simulink library "Library_Betriebsstrategie"  (R2018b)
settings: Solver=VariableStepAuto  StartTime=0.0  StopTime=10.0  RelTol=1e-3  EnableMultiTasking=on
undefined symbols (not defined in the file): akt_eUELG_HA, akt_eUELG_VA, akt_keinMVS_HA, akt_keinMVS_VA, akt_LSD_HA, akt_LSD_VA, akt_mUELG_HA, akt_mUELG_VA, akt_OD_HA, akt_OD_VA, DiscIntNeverNeededParam, magnitude, mu_road, mu_road_LF, mu_road_LR, mu_road_RF, mu_road_RR, par_MDT, par_VEH, stepsize
libraries: simulink x13
(part 4 of 6)

== system Library_Betriebsstrategie/Momentverteilung_LR/Gierrate Referenz Berechnung ==
  note: Gewünschte Gierrate nach:
      | psip_desired = vx * delta / (l + vx^2 * K_us )
  note: Limit für die Gierrate
  input : Inport
  delta_wheel : Inport  Port=2
  FZG parameter : Inport  Port=3
  2 Räder : Constant  Value=0.5
  Abs : Abs
  Abs1 : Abs
  Add : Sum
  Add1 : Sum  Inputs=+--
  Add2 : Sum
  Bus Selector : BusSelector  OutputSignals=l,g
  Bus Selector1 : BusSelector  OutputSignals=delta_RF,delta_LF
  Bus Selector2 : BusSelector  OutputSignals=x.ax,beta.beta,beta.betap,x.vx
  Constant20 : Constant  Value=mu_road
  Divide : Product  Inputs=*/
  Divide1 : Product  Inputs=**/
  Divide2 : Product  Inputs=**/
  Divide3 : Product  Inputs=*/
  Kus : Constant  Value=0
  Product : Product
  Product1 : Product
  Product2 : Product
  Sicherheitsfaktor : Gain  Gain=0.90
  Sign : Signum
  Sqrt : Sqrt  SaturateOnIntegerOverflow=on
  Sum : Sum  Inputs=|++
  delta mittel : Product
  eins : Constant
  min : MinMax  Inputs=2
  tan (beta) : Trigonometry  Operator=tan
  tan^2 (beta) : Math  Operator=square  SaturateOnIntegerOverflow=on
  vx^2 : Math  Operator=square  SaturateOnIntegerOverflow=on
  Gierrate ref : Outport
  wires:
  FZG parameter/1 -> Bus Selector/1
  Product/1 -> Divide/1
  Bus Selector/1 -> Sum/2  "<l>"
  vx^2/1 -> Product1/1
  Sum/1 -> Divide/2
  Product1/1 -> Sum/1
  Kus/1 -> Product1/2
  Divide/1 -> Abs/1  "Gierrate gewuenscht"
  delta_wheel/1 -> Bus Selector1/1
  Bus Selector1/1 -> Add/1  "<delta_RF>"
  Bus Selector1/2 -> Add/2  "<delta_LF>"
  Add/1 -> delta mittel/1
  2 Räder/1 -> delta mittel/2
  delta mittel/1 -> Sign/1, Product/2
  input/1 -> Bus Selector2/1
  Bus Selector2/4 -> Divide2/3, Divide1/3, vx^2/1, Product/1  "<vx>"
  Sicherheitsfaktor/1 -> Abs1/1  "Gierrate Limit"
  Add1/1 -> Sicherheitsfaktor/1
  Sign/1 -> Product2/1  "Vorzeichen von delta"
  min/1 -> Product2/2
  Product2/1 -> Gierrate ref/1
  Abs/1 -> min/1
  Abs1/1 -> min/2
  Divide1/1 -> Add1/1
  Bus Selector/2 -> Divide1/2  "<g>"
  Constant20/1 -> Divide1/1
  Divide2/1 -> Add1/2
  Bus Selector2/1 -> Divide2/2  "<ax>"
  tan (beta)/1 -> tan^2 (beta)/1, Divide2/1
  Bus Selector2/2 -> tan (beta)/1  "<beta>"
  Divide3/1 -> Add1/3
  Bus Selector2/3 -> Divide3/1  "<betap>"
  tan^2 (beta)/1 -> Add2/1
  eins/1 -> Add2/2
  Add2/1 -> Sqrt/1
  Sqrt/1 -> Divide3/2

== system Library_Betriebsstrategie/Momentverteilung_LR/Momente für die Reibbremse ==
  M_antr : Inport
  M_wheel : Inport  Port=2
  v_x : Inport  Port=3
  bkv : Inport  Port=4
  Add : Sum  Inputs=-+
  Add1 : Sum  Inputs=++++
  Bias : Bias  Bias=-1
  Bus Selector : BusSelector  OutputSignals=M_antr_LF,M_antr_LR,M_antr_RF,M_antr_RR
  Product4 : Product  Inputs=3
  Product5 : Product  Inputs=3
  Saturation2 : Saturate  UpperLimit=0  LowerLimit=-5000
  Sign : Signum
  Signal Conversion : SignalConversion  OverrideOpt=off
  Signal Conversion1 : SignalConversion  OverrideOpt=off
  Unary Minus : UnaryMinus
  Unit Delay2 : UnitDelay  InitialCondition=2  SampleTime=-1
  LF : Outport
  LR : Outport  Port=2
  RF : Outport  Port=3
  RR : Outport  Port=4
  wires:
  Add/1 -> Saturation2/1
  Saturation2/1 -> Product5/1, Product4/2
  Bias/1 -> Unary Minus/1
  Unary Minus/1 -> Product5/2
  Signal Conversion/1 -> LF/1  "M_brems_LF"
  Signal Conversion1/1 -> LR/1  "M_brems_LR"
  Product4/1 -> RF/1, Signal Conversion/1  "M_brems_RF"
  Product5/1 -> RR/1, Signal Conversion1/1  "M_brems_RR"
  Sign/1 -> Product4/3, Product5/3
  Unit Delay2/1 -> Sign/1
  bkv/1 -> Product4/1, Bias/1
  v_x/1 -> Unit Delay2/1
  M_wheel/1 -> Add/2
  M_antr/1 -> Bus Selector/1
  Bus Selector/4 -> Add1/4  "<M_antr_RR>"
  Bus Selector/3 -> Add1/3  "<M_antr_RF>"
  Bus Selector/2 -> Add1/2  "<M_antr_LR>"
  Bus Selector/1 -> Add1/1  "<M_antr_LF>"
  Add1/1 -> Add/1

== system Library_Betriebsstrategie/Momentverteilung_LR/Motor Limits ==
  Input : Inport
  Add{1..4} (4 alike) : Sum
  Bus Creator : BusCreator  Inputs=8
  Bus Selector : BusSelector  OutputSignals=omega
  Demux : Demux
  Demux1 : Demux
  Gain{,1..7} (8 alike) : Gain  Gain=0.5
  M_Antr : Lookup_n-D  NumberOfTableDimensions=1  BreakpointsForDimension1=par_VEH.dt_nmax/par_VEH.dt_i/60*2*pi  Table=par_VEH.dt_Mmax*par_VEH.dt_i/2  InternalRulePriority=Speed  RndMeth=Simplest  InputSameDT=on
  M_Reku : Lookup_n-D  NumberOfTableDimensions=1  BreakpointsForDimension1=par_VEH.dt_nmin/par_VEH.dt_i/60*2*pi  Table=par_VEH.dt_Mmin*par_VEH.dt_i/2  InternalRulePriority=Speed  RndMeth=Simplest  InputSameDT=on
  Rate Transition : RateTransition  OutPortSampleTime=stepsize*10
  Rate Transition1 : RateTransition  OutPortSampleTimeOpt=Inherit  OutPortSampleTime=0.001
  Rate Transition2 : RateTransition  OutPortSampleTime=stepsize*10
  Rate Transition3 : RateTransition  OutPortSampleTimeOpt=Inherit  OutPortSampleTime=0.001
  M_limit : Outport
  wires:
  Bus Creator/1 -> M_limit/1
  M_Reku/1 -> Rate Transition1/1
  Rate Transition/1 -> M_Reku/1
  M_Antr/1 -> Rate Transition3/1
  Rate Transition2/1 -> M_Antr/1
  Rate Transition1/1 -> Demux/1
  Demux/1 -> Add1/1
  Demux/2 -> Add1/2
  Add1/1 -> Gain4/1, Gain/1
  Demux/3 -> Add2/1
  Demux/4 -> Add2/2
  Add2/1 -> Gain5/1, Gain1/1
  Demux1/1 -> Add3/1
  Demux1/2 -> Add3/2
  Add3/1 -> Gain6/1, Gain2/1
  Demux1/3 -> Add4/1
  Demux1/4 -> Add4/2
  Add4/1 -> Gain7/1, Gain3/1
  Rate Transition3/1 -> Demux1/1
  Bus Selector/1 -> Rate Transition2/1, Rate Transition/1  "<omega>"
  Input/1 -> Bus Selector/1
  Gain1/1 -> Bus Creator/3  "M_RF_lb"
  Gain2/1 -> Bus Creator/5  "M_LF_ub"
  Gain3/1 -> Bus Creator/7  "M_RF_ub"
  Gain4/1 -> Bus Creator/1  "M_LF_lb"
  Gain/1 -> Bus Creator/2  "M_LR_lb"
  Gain5/1 -> Bus Creator/4  "M_RR_lb"
  Gain6/1 -> Bus Creator/6  "M_LR_ub"
  Gain7/1 -> Bus Creator/8  "M_RR_ub"

== system Library_Betriebsstrategie/Momentverteilung_LR/Radmomentenaufteilung ==
  note: Optimale Distribution Factors
  note: Momentenverteilung
  note: Aufbringen des TV-Moments
  Input : Inport
  M_wheel : Inport  Port=2
  M_z_desired : Inport  Port=3
  FZG parameter : Inport  Port=4
  Bias : Bias  Bias=-1
  Bias1 : Bias  Bias=-1
  Bus Selector : BusSelector  OutputSignals=sF05,r_eff_F
  Divide : Product  Inputs=*/
  Divide1 : Product  Inputs=*/
  Gain : Gain  Gain=0.5
  Optimierung links : Subsystem
  Optimierung rechts : Subsystem
  Product{,1..5} (6 alike) : Product
  Scope2 : Scope  NumInputPorts=4
  Sum : Sum  Inputs=|++
  Sum1 : Sum  Inputs=|+-
  Unary Minus : UnaryMinus
  Unary Minus1 : UnaryMinus
  r_stat0 : Constant  Value=par_VEH.r_stat0
  sF05 : Constant  Value=par_VEH.sF05
  M_antr_LF : Outport
  M_antr_LR : Outport  Port=2
  M_antr_RF : Outport  Port=3
  M_antr_RR : Outport  Port=4
  wires:
  M_wheel/1 -> Divide/1
  M_z_desired/1 -> Divide1/1
  Divide/1 -> Sum1/1, Sum/1  "F_x"
  Divide1/1 -> Sum1/2, Sum/2
  Sum1/1 -> Product/1
  Gain/1 -> Product1/2, Product/2
  Sum/1 -> Product1/1
  Product/1 -> Optimierung links/1(M_wheel_left), Product5/2, Product3/1  "M_wheel_left"
  Product1/1 -> Optimierung rechts/2(M_wheel_right), Product2/1, Product4/2  "M_wheel_right"
  Product3/1 -> Scope2/1, M_antr_LF/1  "M_LF"
  Product4/1 -> M_antr_RR/1, Scope2/4  "M_RR"
  Product5/1 -> Scope2/2, M_antr_LR/1  "M_LR"
  Optimierung rechts/1(gamma_right) -> Bias1/1, Product2/2
  r_stat0/1 -> Divide/2, Gain/1
  sF05/1 -> Divide1/2
  Product2/1 -> Scope2/3, M_antr_RF/1  "M_RF"
  Input/1 -> Optimierung links/2(Input), Optimierung rechts/1(Input)
  FZG parameter/1 -> Bus Selector/1
  Bias/1 -> Unary Minus/1
  Optimierung links/1(gamma_left) -> Bias/1, Product3/2
  Unary Minus/1 -> Product5/1
  Bias1/1 -> Unary Minus1/1
  Unary Minus1/1 -> Product4/1

== system Library_Betriebsstrategie/Momentverteilung_LR/Reifen Limits ==
  note: Kammscher Kreis liefert mit aktuellen mue und F_z_i die limits für Fx
  ParVehicle : Inport
  Fx_limits : Outport

== system Library_Betriebsstrategie/Momentverteilung_LR1/Feedback Controller ==
  note: Sigmoid Funktion
  note: M_z punkt = - Iz * K * sign(sigma - 1/2sigma(Tc))
  note: 1/2 sigma(Tc)
  Gierrate : Inport
  Gierrate ref : Inport  Port=2
  Iz : Inport  Port=3
  -1 : Gain  Gain=-1
  Abs : Abs
  Add : Sum
  Discrete D : simulink/Discrete/Discrete Derivative  gainval=1.0  ICPrevScaledInput=0.0  OutMin=[]  OutMax=[]  OutDataType=fixdt(1, 16)  OutScaling=2^-10  DoSatur=off
  Discrete-Time Integrator : DiscreteIntegrator  SampleTime=0.1  ICPrevOutput=DiscIntNeverNeededParam  ICPrevScaledInput=DiscIntNeverNeededParam
  Divide : Product  Inputs=*/
  Divide1 : Product  Inputs=*/
  Einheitenkorrektur : Constant  Value=1000
  Gain : Gain  Gain=0.5
  K : Gain  Gain=8
  Memory : Memory  LinearizeAsDelay=on
  Product : Product
  Sum : Sum  Inputs=|-+
  Sum1 : Sum  Inputs=|+-
  Unit Delay : UnitDelay  SampleTime=0.1
  Zero Crossing : Subsystem
  epsilon : Constant  Value=0.015
  M_z_desired : Outport
  wires:
  Divide1/1 -> Product/2
  Einheitenkorrektur/1 -> Divide1/2
  Iz/1 -> Divide1/1
  Zero Crossing/1(error(Tc)) -> Gain/1, Memory/1
  Unit Delay/1 -> Zero Crossing/2(de1)
  Memory/1 -> Zero Crossing/4(e1)
  Gain/1 -> Sum1/2
  Discrete D/1 -> Unit Delay/1, Zero Crossing/1(de0)
  Discrete-Time Integrator/1 -> M_z_desired/1
  -1/1 -> Discrete-Time Integrator/1
  Product/1 -> -1/1
  K/1 -> Product/1
  Divide/1 -> K/1
  Add/1 -> Divide/2
  epsilon/1 -> Add/2
  Abs/1 -> Add/1
  Sum1/1 -> Abs/1, Divide/1
  Sum/1 -> Discrete D/1, Zero Crossing/3(e0), Sum1/1  "sigma = - error"
  Gierrate ref/1 -> Sum/1
  Gierrate/1 -> Sum/2

== system Library_Betriebsstrategie/Momentverteilung_LR1/Gierrate Referenz Berechnung ==
  note: Limit für die Gierrate
  note: Gewünschte Gierrate nach:
      | psip_desired = vx * delta / (l + vx^2 * K_us )
  input : Inport
  delta_wheel : Inport  Port=2
  FZG parameter : Inport  Port=3
  2 Räder : Constant  Value=0.5
  Abs : Abs
  Abs1 : Abs
  Add : Sum
  Add1 : Sum  Inputs=+--
  Add2 : Sum
  Bus Selector : BusSelector  OutputSignals=l,g
  Bus Selector1 : BusSelector  OutputSignals=delta_RF,delta_LF
  Bus Selector2 : BusSelector  OutputSignals=x.ax,beta.beta,beta.betap,x.vx
  Constant20 : Constant  Value=mu_road
  Divide : Product  Inputs=*/
  Divide1 : Product  Inputs=**/
  Divide2 : Product  Inputs=**/
  Divide3 : Product  Inputs=*/
  Kus : Constant  Value=0
  Product : Product
  Product1 : Product
  Product2 : Product
  Sicherheitsfaktor : Gain  Gain=0.90
  Sign : Signum
  Sqrt : Sqrt  SaturateOnIntegerOverflow=on
  Sum : Sum  Inputs=|++
  delta mittel : Product
  eins : Constant
  min : MinMax  Inputs=2
  tan (beta) : Trigonometry  Operator=tan
  tan^2 (beta) : Math  Operator=square  SaturateOnIntegerOverflow=on
  vx^2 : Math  Operator=square  SaturateOnIntegerOverflow=on
  Gierrate ref : Outport
  wires:
  Sqrt/1 -> Divide3/2
  Add2/1 -> Sqrt/1
  eins/1 -> Add2/2
  tan^2 (beta)/1 -> Add2/1
  Bus Selector2/3 -> Divide3/1  "<betap>"
  Divide3/1 -> Add1/3
  Bus Selector2/2 -> tan (beta)/1  "<beta>"
  tan (beta)/1 -> Divide2/1, tan^2 (beta)/1
  Bus Selector2/1 -> Divide2/2  "<ax>"
  Divide2/1 -> Add1/2
  Constant20/1 -> Divide1/1
  Bus Selector/2 -> Divide1/2  "<g>"
  Divide1/1 -> Add1/1
  Abs1/1 -> min/2
  Abs/1 -> min/1
  Product2/1 -> Gierrate ref/1
  min/1 -> Product2/2
  Sign/1 -> Product2/1  "Vorzeichen von delta"
  Add1/1 -> Sicherheitsfaktor/1
  Sicherheitsfaktor/1 -> Abs1/1  "Gierrate Limit"
  Bus Selector2/4 -> Product/1, vx^2/1, Divide1/3, Divide2/3  "<vx>"
  input/1 -> Bus Selector2/1
  delta mittel/1 -> Product/2, Sign/1
  2 Räder/1 -> delta mittel/2
  Add/1 -> delta mittel/1
  Bus Selector1/2 -> Add/2  "<delta_LF>"
  Bus Selector1/1 -> Add/1  "<delta_RF>"
  delta_wheel/1 -> Bus Selector1/1
  Divide/1 -> Abs/1  "Gierrate gewuenscht"
  Kus/1 -> Product1/2
  Product1/1 -> Sum/1
  Sum/1 -> Divide/2
  vx^2/1 -> Product1/1
  Bus Selector/1 -> Sum/2  "<l>"
  Product/1 -> Divide/1
  FZG parameter/1 -> Bus Selector/1

== system Library_Betriebsstrategie/Momentverteilung_LR1/Limitierungen gesamt ==
  Fx_limit : Inport
  M_limit : Inport  Port=2
  MVS_limit : Inport  Port=3
  Bus Creator : BusCreator  Inputs=8
  Bus Selector : BusSelector  OutputSignals=FxlimFR,FxlimFL,FxlimRR,FxlimRL
  Bus Selector1 : BusSelector  OutputSignals=M_RF_ub,M_RF_lb,M_LF_ub,M_LF_lb,M_RR_ub,M_RR_lb,M_LR_ub,M_LR_lb
  Divide{,1..7} (8 alike) : Product  Inputs=*/
  Gain{,1..3} (4 alike) : Gain  Gain=-1
  Max_FL : MinMax  Function=max  Inputs=2
  Max_FR : MinMax  Function=max  Inputs=2
  Max_FR1 : MinMax  Function=max  Inputs=2
  Max_RR : MinMax  Function=max  Inputs=2
  Min_FL : MinMax  Inputs=2
  Min_FR : MinMax  Inputs=2
  Min_FR1 : MinMax  Inputs=2
  Min_RR : MinMax  Inputs=2
  r_stat{0..7} (8 alike) : Constant  Value=par_VEH.r_stat0
  Fx_limits : Outport
  wires:
  Fx_limit/1 -> Bus Selector/1
  M_limit/1 -> Bus Selector1/1
  Bus Selector1/1 -> Divide/1  "<M_RF_ub>"
  Bus Selector/1 -> Gain/1, Min_FR/1  "<FxlimFR>"
  r_stat0/1 -> Divide/2
  Divide/1 -> Min_FR/2
  Bus Creator/1 -> Fx_limits/1
  Min_FR/1 -> Bus Creator/1  "Fx_FR_ub"
  Bus Selector1/2 -> Divide1/1  "<M_RF_lb>"
  r_stat1/1 -> Divide1/2
  Divide1/1 -> Max_FR/2
  Gain/1 -> Max_FR/1
  Max_FR/1 -> Bus Creator/2  "Fx_FR_lb"
  r_stat2/1 -> Divide2/2
  Divide2/1 -> Min_FL/2
  r_stat3/1 -> Divide3/2
  Divide3/1 -> Max_FL/2
  Gain1/1 -> Max_FL/1
  Bus Selector/2 -> Gain1/1, Min_FL/1  "<FxlimFL>"
  Bus Selector1/3 -> Divide2/1  "<M_LF_ub>"
  Bus Selector1/4 -> Divide3/1  "<M_LF_lb>"
  Min_FL/1 -> Bus Creator/3  "Fx_FL_ub"
  Max_FL/1 -> Bus Creator/4  "Fx_FL_lb"
  r_stat4/1 -> Divide4/2
  Divide4/1 -> Min_RR/2
  Min_RR/1 -> Bus Creator/5  "Fx_RR_ub"
  r_stat5/1 -> Divide5/2
  Divide5/1 -> Max_RR/2
  Gain2/1 -> Max_RR/1
  Max_RR/1 -> Bus Creator/6  "Fx_RR_lb"
  Bus Selector1/5 -> Divide4/1  "<M_RR_ub>"
  Bus Selector1/6 -> Divide5/1  "<M_RR_lb>"
  Bus Selector/3 -> Gain2/1, Min_RR/1  "<FxlimRR>"
  r_stat6/1 -> Divide6/2
  Divide6/1 -> Min_FR1/2
  Min_FR1/1 -> Bus Creator/7  "Fx_RL_ub"
  r_stat7/1 -> Divide7/2
  Divide7/1 -> Max_FR1/2
  Gain3/1 -> Max_FR1/1
  Max_FR1/1 -> Bus Creator/8  "Fx_RL_lb"
  Bus Selector1/7 -> Divide6/1  "<M_LR_ub>"
  Bus Selector1/8 -> Divide7/1  "<M_LR_lb>"
  Bus Selector/4 -> Gain3/1, Min_FR1/1  "<FxlimRL>"

== system Library_Betriebsstrategie/Momentverteilung_LR1/Momente für die Reibbremse ==
  M_antr : Inport
  M_wheel : Inport  Port=2
  v_x : Inport  Port=3
  bkv : Inport  Port=4
  Add : Sum  Inputs=-+
  Add1 : Sum  Inputs=++++
  Bias : Bias  Bias=-1
  Bus Selector : BusSelector  OutputSignals=M_antr_LF,M_antr_LR,M_antr_RF,M_antr_RR
  Product4 : Product  Inputs=3
  Product5 : Product  Inputs=3
  Saturation2 : Saturate  UpperLimit=0  LowerLimit=-5000
  Sign : Signum
  Signal Conversion : SignalConversion  OverrideOpt=off
  Signal Conversion1 : SignalConversion  OverrideOpt=off
  Unary Minus : UnaryMinus
  Unit Delay2 : UnitDelay  InitialCondition=2  SampleTime=-1
  LF : Outport
  LR : Outport  Port=2
  RF : Outport  Port=3
  RR : Outport  Port=4
  wires:
  Add1/1 -> Add/1
  Bus Selector/1 -> Add1/1  "<M_antr_LF>"
  Bus Selector/2 -> Add1/2  "<M_antr_LR>"
  Bus Selector/3 -> Add1/3  "<M_antr_RF>"
  Bus Selector/4 -> Add1/4  "<M_antr_RR>"
  M_antr/1 -> Bus Selector/1
  M_wheel/1 -> Add/2
  v_x/1 -> Unit Delay2/1
  bkv/1 -> Bias/1, Product4/1
  Unit Delay2/1 -> Sign/1
  Sign/1 -> Product5/3, Product4/3
  Product5/1 -> Signal Conversion1/1, RR/1  "M_brems_RR"
  Product4/1 -> Signal Conversion/1, RF/1  "M_brems_RF"
  Signal Conversion1/1 -> LR/1  "M_brems_LR"
  Signal Conversion/1 -> LF/1  "M_brems_LF"
  Unary Minus/1 -> Product5/2
  Bias/1 -> Unary Minus/1
  Saturation2/1 -> Product4/2, Product5/1
  Add/1 -> Saturation2/1

== system Library_Betriebsstrategie/Momentverteilung_LR1/Momentenverteilende Systeme Limits ==
  Input : Inport
  MVS_limit : Outport
  wires:
  Input/1 -> MVS_limit/1

== system Library_Betriebsstrategie/Momentverteilung_LR1/Motor Limits ==
  Input : Inport
  Add{1..4} (4 alike) : Sum
  Bus Creator : BusCreator  Inputs=8
  Bus Selector : BusSelector  OutputSignals=omega
  Demux : Demux
  Demux1 : Demux
  Gain{,1..7} (8 alike) : Gain  Gain=0.5
  M_Antr : Lookup_n-D  NumberOfTableDimensions=1  BreakpointsForDimension1=par_VEH.dt_nmax/par_VEH.dt_i/60*2*pi  Table=par_VEH.dt_Mmax*par_VEH.dt_i/2  InternalRulePriority=Speed  RndMeth=Simplest  InputSameDT=on
  M_Reku : Lookup_n-D  NumberOfTableDimensions=1  BreakpointsForDimension1=par_VEH.dt_nmin/par_VEH.dt_i/60*2*pi  Table=par_VEH.dt_Mmin*par_VEH.dt_i/2  InternalRulePriority=Speed  RndMeth=Simplest  InputSameDT=on
  Rate Transition : RateTransition  OutPortSampleTime=stepsize*10
  Rate Transition1 : RateTransition  OutPortSampleTimeOpt=Inherit  OutPortSampleTime=0.001
  Rate Transition2 : RateTransition  OutPortSampleTime=stepsize*10
  Rate Transition3 : RateTransition  OutPortSampleTimeOpt=Inherit  OutPortSampleTime=0.001
  M_limit : Outport
  wires:
  Gain7/1 -> Bus Creator/8  "M_RR_ub"
  Gain6/1 -> Bus Creator/6  "M_LR_ub"
  Gain5/1 -> Bus Creator/4  "M_RR_lb"
  Gain/1 -> Bus Creator/2  "M_LR_lb"
  Gain4/1 -> Bus Creator/1  "M_LF_lb"
  Gain3/1 -> Bus Creator/7  "M_RF_ub"
  Gain2/1 -> Bus Creator/5  "M_LF_ub"
  Gain1/1 -> Bus Creator/3  "M_RF_lb"
  Input/1 -> Bus Selector/1
  Bus Selector/1 -> Rate Transition2/1, Rate Transition/1  "<omega>"
  Rate Transition3/1 -> Demux1/1
  Add4/1 -> Gain3/1, Gain7/1
  Demux1/4 -> Add4/2
  Demux1/3 -> Add4/1
  Add3/1 -> Gain2/1, Gain6/1
  Demux1/2 -> Add3/2
  Demux1/1 -> Add3/1
  Add2/1 -> Gain1/1, Gain5/1
  Demux/4 -> Add2/2
  Demux/3 -> Add2/1
  Add1/1 -> Gain/1, Gain4/1
  Demux/2 -> Add1/2
  Demux/1 -> Add1/1
  Rate Transition1/1 -> Demux/1
  Rate Transition2/1 -> M_Antr/1
  M_Antr/1 -> Rate Transition3/1
  Rate Transition/1 -> M_Reku/1
  M_Reku/1 -> Rate Transition1/1
  Bus Creator/1 -> M_limit/1

== system Library_Betriebsstrategie/Momentverteilung_LR1/Radmomentenaufteilung ==
  note: Aufbringen des TV-Moments
  note: Momentenverteilung
  note: Optimale Distribution Factors
  Input : Inport
  M_wheel : Inport  Port=2
  M_z_desired : Inport  Port=3
  FZG parameter : Inport  Port=4
  Bias : Bias  Bias=-1
  Bias1 : Bias  Bias=-1
  Bus Selector : BusSelector  OutputSignals=sF05,r_eff_F
  Divide : Product  Inputs=*/
  Divide1 : Product  Inputs=*/
  Gain : Gain  Gain=0.5
  Optimierung links : Subsystem
  Optimierung rechts : Subsystem
  Product{,1..5} (6 alike) : Product
  Scope2 : Scope  NumInputPorts=4
  Sum : Sum  Inputs=|++
  Sum1 : Sum  Inputs=|+-
  Unary Minus : UnaryMinus
  Unary Minus1 : UnaryMinus
  r_stat0 : Constant  Value=par_VEH.r_stat0
  sF05 : Constant  Value=par_VEH.sF05
  M_antr_LF : Outport
  M_antr_LR : Outport  Port=2
  M_antr_RF : Outport  Port=3
  M_antr_RR : Outport  Port=4
  wires:
  Unary Minus1/1 -> Product4/1
  Bias1/1 -> Unary Minus1/1
  Unary Minus/1 -> Product5/1
  Optimierung links/1(gamma_left) -> Product3/2, Bias/1
  Bias/1 -> Unary Minus/1
  FZG parameter/1 -> Bus Selector/1
  Input/1 -> Optimierung rechts/1(Input), Optimierung links/2(Input)
  Product2/1 -> M_antr_RF/1, Scope2/3  "M_RF"
  sF05/1 -> Divide1/2
  r_stat0/1 -> Gain/1, Divide/2
  Optimierung rechts/1(gamma_right) -> Product2/2, Bias1/1
  Product5/1 -> M_antr_LR/1, Scope2/2  "M_LR"
  Product4/1 -> Scope2/4, M_antr_RR/1  "M_RR"
  Product3/1 -> M_antr_LF/1, Scope2/1  "M_LF"
  Product1/1 -> Product4/2, Product2/1, Optimierung rechts/2(M_wheel_right)  "M_wheel_right"
  Product/1 -> Product3/1, Product5/2, Optimierung links/1(M_wheel_left)  "M_wheel_left"
  Sum/1 -> Product1/1
  Gain/1 -> Product/2, Product1/2
  Sum1/1 -> Product/1
  Divide1/1 -> Sum/2, Sum1/2
  Divide/1 -> Sum/1, Sum1/1  "F_x"
  M_z_desired/1 -> Divide1/1
  M_wheel/1 -> Divide/1

== system Library_Betriebsstrategie/Momentverteilung_LR1/Reifen Limits ==
  Input : Inport
  Add{,1..3} (4 alike) : Sum  Inputs=-+
  Bus Creator : BusCreator  Inputs=4
  Bus Selector1 : BusSelector  OutputSignals=Fz.Fz_RF,Fs.Fs_RF,Fz.Fz_LF,Fs.Fs_LF,Fz.Fz_RR,Fs.Fs_RR,Fz.Fz_LR,Fs.Fs_LR
  Constant{,1..3} (4 alike) : Constant
  Constant20 : Constant  Value=mu_road
  Divide{,1..3} (4 alike) : Product  Inputs=/*
  Math Function{,1..3} (4 alike) : Math  Operator=magnitude^2  SaturateOnIntegerOverflow=on
  Product{,1..11} (12 alike) : Product
  Scope{3..5,9,11} (5 alike) : Scope
  Sqrt{,1..3} (4 alike) : Sqrt  SaturateOnIntegerOverflow=on
  Fx_limit : Outport
  wires:
  Bus Creator/1 -> Fx_limit/1
  Product3/1 -> Bus Creator/4  "FxlimRL"
  Product1/1 -> Bus Creator/3  "FxlimRR"
  Product2/1 -> Bus Creator/2  "FxlimFL"
  Product/1 -> Bus Creator/1  "FxlimFR"
  Bus Selector1/8 -> Divide3/2  "<Fs_LR>"
  Bus Selector1/6 -> Divide1/2  "<Fs_RR>"
  Bus Selector1/4 -> Divide2/2, Scope11/1  "<Fs_LF>"
  Bus Selector1/2 -> Divide/2  "<Fs_RF>"
  Bus Selector1/7 -> Product10/2, Product11/2  "<Fz_LR>"
  Bus Selector1/5 -> Product8/2, Product9/2  "<Fz_RR>"
  Bus Selector1/3 -> Product6/2, Product7/2  "<Fz_LF>"
  Bus Selector1/1 -> Product4/2, Product5/2  "<Fz_RF>"
  Constant20/1 -> Product4/1, Product5/1, Product6/1, Product7/1, Product10/1, Product11/1, Product8/1, Product9/1  "mu_road"
  Input/1 -> Bus Selector1/1
  Divide/1 -> Math Function/1
  Sqrt3/1 -> Product3/2
  Add3/1 -> Sqrt3/1
  Constant3/1 -> Add3/2
  Math Function3/1 -> Add3/1
  Divide3/1 -> Math Function3/1, Scope5/1
  Product11/1 -> Divide3/1, Scope9/1
  Product10/1 -> Product3/1
  Sqrt2/1 -> Product2/2
  Add2/1 -> Sqrt2/1
  Constant2/1 -> Add2/2
  Math Function2/1 -> Add2/1
  Divide2/1 -> Math Function2/1
  Product7/1 -> Divide2/1, Scope3/1
  Product6/1 -> Product2/1
  Sqrt1/1 -> Product1/2
  Add1/1 -> Sqrt1/1
  Constant1/1 -> Add1/2
  Math Function1/1 -> Add1/1
  Divide1/1 -> Math Function1/1, Scope4/1
  Product9/1 -> Divide1/1
  Product8/1 -> Product1/1
  Sqrt/1 -> Product/2
  Add/1 -> Sqrt/1
  Constant/1 -> Add/2
  Math Function/1 -> Add/1
  Product5/1 -> Divide/1
  Product4/1 -> Product/1

== system Library_Betriebsstrategie/Momentverteilung_LR2/Feedback Controller ==
  note: 1/2 sigma(Tc)
  note: M_z punkt = - Iz * K * sign(sigma - 1/2sigma(Tc))
  note: Sigmoid Funktion
  Gierrate : Inport
  Gierrate ref : Inport  Port=2
  -1 : Gain  Gain=-1
  Abs : Abs
  Add : Sum
  Bus to Vector1 : BusToVector
  Bus to Vector18 : BusToVector
  Bus to Vector2 : BusToVector
  Constant10 : Constant  Value=par_VEH.Iz
  Discrete D : simulink/Discrete/Discrete Derivative  gainval=1.0  ICPrevScaledInput=0.0  OutMin=[]  OutMax=[]  OutDataType=fixdt(1, 16)  OutScaling=2^-10  DoSatur=off
  Discrete-Time Integrator : DiscreteIntegrator  SampleTime=-1  ICPrevOutput=DiscIntNeverNeededParam  ICPrevScaledInput=DiscIntNeverNeededParam
  Divide : Product  Inputs=*/
  Divide1 : Product  Inputs=*/
  Einheitenkorrektur : Constant  Value=1000
  Gain : Gain  Gain=0.5
  K : Gain  Gain=8
  Memory : Memory  LinearizeAsDelay=on
  Product : Product
  Sum : Sum  Inputs=|-+
  Sum1 : Sum  Inputs=|+-
  To Workspace1 : ToWorkspace  VariableName=sv_psiP  SampleTime=-1
      settings: Decimation=savedec  Save2DSignal=2-D array (concatenate along first dimension)
  To Workspace2 : ToWorkspace  VariableName=sv_Mz_des  SampleTime=-1
      settings: Decimation=savedec  Save2DSignal=2-D array (concatenate along first dimension)
  To Workspace32 : ToWorkspace  VariableName=sv_psiP_ref  SampleTime=-1
      settings: Decimation=savedec  Save2DSignal=2-D array (concatenate along first dimension)
  Unit Delay : UnitDelay  SampleTime=-1
  Zero Crossing : Subsystem
  epsilon : Constant  Value=0.015
  M_z_desired : Outport
  wires:
  Sum/1 -> Sum1/1, Zero Crossing/3(e0), Discrete D/1  "sigma = - error"
  Sum1/1 -> Divide/1, Abs/1
  Abs/1 -> Add/1
  epsilon/1 -> Add/2
  Add/1 -> Divide/2
  Divide/1 -> K/1
  K/1 -> Product/1
  Product/1 -> -1/1
  -1/1 -> Discrete-Time Integrator/1
  Discrete D/1 -> Zero Crossing/1(de0), Unit Delay/1
  Gain/1 -> Sum1/2
  Memory/1 -> Zero Crossing/4(e1)
  Unit Delay/1 -> Zero Crossing/2(de1)
  Zero Crossing/1(error(Tc)) -> Memory/1, Gain/1
  Einheitenkorrektur/1 -> Divide1/2
  Divide1/1 -> Product/2
  Bus to Vector18/1 -> To Workspace32/1
  Gierrate ref/1 -> Bus to Vector18/1, Sum/1
  Bus to Vector1/1 -> To Workspace1/1
  Gierrate/1 -> Bus to Vector1/1, Sum/2
  Bus to Vector2/1 -> To Workspace2/1
  Discrete-Time Integrator/1 -> Bus to Vector2/1, M_z_desired/1
  Constant10/1 -> Divide1/1

== system Library_Betriebsstrategie/Momentverteilung_LR2/Gierrate Referenz Berechnung ==
  note: Gewünschte Gierrate nach:
      | psip_desired = vx * delta / (l + vx^2 * K_us )
  note: Limit für die Gierrate
  input : Inport
  delta_wheel : Inport  Port=2
  2 Räder : Constant  Value=0.5
  Abs : Abs
  Abs1 : Abs
  Add : Sum
  Add1 : Sum  Inputs=+--
  Add2 : Sum
  Bus Selector1 : BusSelector  OutputSignals=delta_RF,delta_LF
  Bus Selector2 : BusSelector  OutputSignals=x.ax,beta.beta,beta.betap,x.vx
  Constant1 : Constant  Value=par_VEH.g
  Constant10 : Constant  Value=par_VEH.l
  Constant20 : Constant  Value=mu_road
  Divide : Product  Inputs=*/
  Divide1 : Product  Inputs=**/
  Divide2 : Product  Inputs=**/
  Divide3 : Product  Inputs=*/
  Kus : Constant  Value=0
  Product : Product
  Product1 : Product
  Product2 : Product
  Sicherheitsfaktor : Gain  Gain=0.90
  Sign : Signum
  Sqrt : Sqrt  SaturateOnIntegerOverflow=on
  Sum : Sum  Inputs=|++
  Sum1 : Sum  Inputs=|++
  delta mittel : Product
  eins : Constant
  epsilon : Constant  Value=0.0015
  min : MinMax  Inputs=2
  tan (beta)1 : Trigonometry  Operator=tan
  tan^2 (beta)1 : Math  Operator=square  SaturateOnIntegerOverflow=on
  vx^2 : Math  Operator=square  SaturateOnIntegerOverflow=on
  Gierrate ref : Outport
  wires:
  Product/1 -> Divide/1
  Constant10/1 -> Sum/2
  vx^2/1 -> Product1/1
  Sum/1 -> Divide/2
  Product1/1 -> Sum/1
  Kus/1 -> Product1/2
  Divide/1 -> Abs/1  "Gierrate gewuenscht"
  delta_wheel/1 -> Bus Selector1/1
  Bus Selector1/1 -> Add/1  "<delta_RF>"
  Bus Selector1/2 -> Add/2  "<delta_LF>"
  Add/1 -> delta mittel/1
  2 Räder/1 -> delta mittel/2
  delta mittel/1 -> Sign/1, Product/2
  input/1 -> Bus Selector2/1
  Bus Selector2/4 -> Sum1/1, vx^2/1, Product/1  "<vx>"
  Sicherheitsfaktor/1 -> Abs1/1  "Gierrate Limit"
  Add1/1 -> Sicherheitsfaktor/1
  Sign/1 -> Product2/1  "Vorzeichen von delta"
  min/1 -> Product2/2
  Product2/1 -> Gierrate ref/1
  Abs/1 -> min/1
  Abs1/1 -> min/2
  Divide1/1 -> Add1/1
  Constant1/1 -> Divide1/2
  Constant20/1 -> Divide1/1
  Divide2/1 -> Add1/2
  Bus Selector2/1 -> Divide2/2  "<ax>"
  tan (beta)1/1 -> tan^2 (beta)1/1, Divide2/1
  Bus Selector2/2 -> tan (beta)1/1  "<beta>"
  Divide3/1 -> Add1/3
  Bus Selector2/3 -> Divide3/1  "<betap>"
  tan^2 (beta)1/1 -> Add2/1
  eins/1 -> Add2/2
  Add2/1 -> Sqrt/1
  Sqrt/1 -> Divide3/2
  Sum1/1 -> Divide2/3, Divide1/3
  epsilon/1 -> Sum1/2

== system Library_Betriebsstrategie/Momentverteilung_LR2/Limitierungen gesamt (mit MVS Limits) ==
  Fx_limit : Inport
  M_limit : Inport  Port=2
  M_limit_zentral : Inport  Port=3
  Bus Creator : BusCreator  Inputs=8
  Bus Selector : BusSelector  OutputSignals=FxlimRF,FxlimLF,FxlimRR,FxlimLR
  Bus Selector1 : BusSelector  OutputSignals=M_RF_ub,M_RF_lb,M_LF_ub,M_LF_lb,M_RR_ub,M_RR_lb,M_LR_ub,M_LR_lb
  Bus Selector2 : BusSelector  OutputSignals=M_F_lb,M_F_ub,M_R_lb,M_R_ub
  Limits Zusammenführung : MATLAB Function  TreatAsAtomicUnit=on
  Subsystem : Subsystem
  a_f : Constant
  a_r : Constant
  r_stat0 : Constant  Value=par_VEH.r_stat0
  Fx_limits : Outport
  wires:
  Bus Selector2/4 -> Limits Zusammenführung/16(M_R_ub)  "<M_R_ub>"
  Bus Selector2/3 -> Limits Zusammenführung/15(M_R_lb)  "<M_R_lb>"
  Bus Selector2/2 -> Limits Zusammenführung/14(M_F_ub)  "<M_F_ub>"
  Bus Selector2/1 -> Limits Zusammenführung/13(M_F_lb)  "<M_F_lb>"
  M_limit_zentral/1 -> Bus Selector2/1
  Bus Selector1/8 -> Limits Zusammenführung/12(M_LR_lb)  "<M_LR_lb>"
  Bus Selector1/7 -> Limits Zusammenführung/11(M_LR_ub)  "<M_LR_ub>"
  Bus Selector1/6 -> Limits Zusammenführung/10(M_RR_lb)  "<M_RR_lb>"
  Bus Selector1/5 -> Limits Zusammenführung/9(M_RR_ub)  "<M_RR_ub>"
  Bus Selector1/4 -> Limits Zusammenführung/8(M_LF_lb)  "<M_LF_lb>"
  Bus Selector1/3 -> Limits Zusammenführung/7(M_LF_ub)  "<M_LF_ub>"
  Bus Selector1/2 -> Limits Zusammenführung/6(M_RF_lb)  "<M_RF_lb>"
  Bus Selector1/1 -> Limits Zusammenführung/5(M_RF_ub)  "<M_RF_ub>"
  Bus Selector/4 -> Limits Zusammenführung/4(FxlimLR)  "<FxlimLR>"
  Bus Selector/3 -> Limits Zusammenführung/3(FxlimRR)  "<FxlimRR>"
  Bus Selector/2 -> Limits Zusammenführung/2(FxlimLF)  "<FxlimLF>"
  Bus Selector/1 -> Limits Zusammenführung/1(FxlimRF)  "<FxlimRF>"
  Bus Creator/1 -> Fx_limits/1
  M_limit/1 -> Bus Selector1/1
  Fx_limit/1 -> Bus Selector/1
  r_stat0/1 -> Limits Zusammenführung/21(r)
  Subsystem/1(Delta_T_f) -> Limits Zusammenführung/17(DELTA_T_f)
  Subsystem/2(Delta_T_r) -> Limits Zusammenführung/18(DELTA_T_r)
  a_f/1 -> Limits Zusammenführung/19(a_f), Subsystem/1(a_f)
  a_r/1 -> Limits Zusammenführung/20(a_r), Subsystem/2(a_r)
  Limits Zusammenführung/1(Fx_LF_ub) -> Bus Creator/1  "Fx_LF_ub"
  Limits Zusammenführung/2(Fx_LF_lb) -> Bus Creator/2  "Fx_LF_lb"
  Limits Zusammenführung/3(Fx_RF_ub) -> Bus Creator/3  "Fx_RF_ub"
  Limits Zusammenführung/4(Fx_RF_lb) -> Bus Creator/4  "Fx_RF_lb"
  Limits Zusammenführung/5(Fx_LR_ub) -> Bus Creator/5  "Fx_LR_ub"
  Limits Zusammenführung/6(Fx_LR_lb) -> Bus Creator/6  "Fx_LR_lb"
  Limits Zusammenführung/7(Fx_RR_ub) -> Bus Creator/7  "Fx_RR_ub"
  Limits Zusammenführung/8(Fx_RR_lb) -> Bus Creator/8  "Fx_RR_lb"

== system Library_Betriebsstrategie/Momentverteilung_LR2/Momente für die Reibbremse ==
  M_antr : Inport
  M_wheel : Inport  Port=2
  v_x : Inport  Port=3
  bkv : Inport  Port=4
  Add : Sum  Inputs=-+
  Add1 : Sum  Inputs=++++
  Bias : Bias  Bias=-1
  Bus Selector : BusSelector  OutputSignals=M_antr_LF,M_antr_LR,M_antr_RF,M_antr_RR
  Product4 : Product  Inputs=3
  Product5 : Product  Inputs=3
  Saturation2 : Saturate  UpperLimit=0  LowerLimit=-5000
  Sign : Signum
  Signal Conversion : SignalConversion  OverrideOpt=off
  Signal Conversion1 : SignalConversion  OverrideOpt=off
  To Workspace4 : ToWorkspace  VariableName=sv_M_Bremse  SampleTime=-1
      settings: Decimation=savedec  Save2DSignal=2-D array (concatenate along first dimension)
  Unary Minus : UnaryMinus
  Unit Delay2 : UnitDelay  InitialCondition=2  SampleTime=-1
  LF : Outport
  LR : Outport  Port=2
  RF : Outport  Port=3
  RR : Outport  Port=4
  wires:
  Add/1 -> Saturation2/1, To Workspace4/1
  Saturation2/1 -> Product5/1, Product4/2
  Bias/1 -> Unary Minus/1
  Unary Minus/1 -> Product5/2
  Signal Conversion/1 -> LF/1  "M_brems_LF"
  Signal Conversion1/1 -> LR/1  "M_brems_LR"
  Product4/1 -> RF/1, Signal Conversion/1  "M_brems_RF"
  Product5/1 -> RR/1, Signal Conversion1/1  "M_brems_RR"
  Sign/1 -> Product4/3, Product5/3
  Unit Delay2/1 -> Sign/1
  bkv/1 -> Product4/1, Bias/1
  v_x/1 -> Unit Delay2/1
  M_wheel/1 -> Add/2
  M_antr/1 -> Bus Selector/1
  Bus Selector/4 -> Add1/4  "<M_antr_RR>"
  Bus Selector/3 -> Add1/3  "<M_antr_RF>"
  Bus Selector/2 -> Add1/2  "<M_antr_LR>"
  Bus Selector/1 -> Add1/1  "<M_antr_LF>"
  Add1/1 -> Add/1

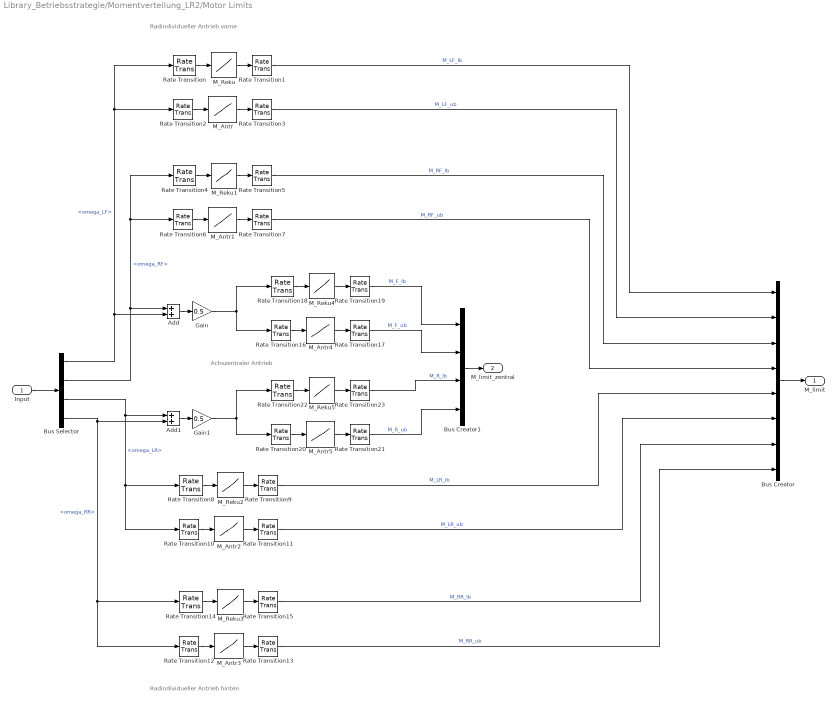
== system Library_Betriebsstrategie/Momentverteilung_LR2/Motor Limits ==
  note: Radindividueller Antrieb vorne
  note: Radindividueller Antrieb hinten
  note: Achszentraler Antrieb
  Input : Inport
  Add : Sum
  Add1 : Sum
  Bus Creator : BusCreator  Inputs=8
  Bus Creator1 : BusCreator  Inputs=4
  Bus Selector : BusSelector  OutputSignals=omega.omega_LF,omega.omega_RF,omega.omega_LR,omega.omega_RR
  Gain : Gain  Gain=0.5
  Gain1 : Gain  Gain=0.5
  M_Antr{,1..5} (6 alike) : Lookup_n-D  NumberOfTableDimensions=1  BreakpointsForDimension1=par_VEH.dt_nmax/par_VEH.dt_i/60*2*pi  Table=par_VEH.dt_Mmax*par_VEH.dt_i/2  InternalRulePriority=Speed  RndMeth=Simplest  InputSameDT=on
  M_Reku{,1..5} (6 alike) : Lookup_n-D  NumberOfTableDimensions=1  BreakpointsForDimension1=par_VEH.dt_nmin/par_VEH.dt_i/60*2*pi  Table=par_VEH.dt_Mmin*par_VEH.dt_i/2  InternalRulePriority=Speed  RndMeth=Simplest  InputSameDT=on
  Rate Transition{,2,4,6,8,10,12,14,16,18,20,22} (12 alike) : RateTransition  OutPortSampleTime=stepsize*10
  Rate Transition{1,3,5,7,9,11,13,15,17,19,21,23} (12 alike) : RateTransition  OutPortSampleTimeOpt=Inherit  OutPortSampleTime=0.001
  M_limit : Outport
  M_limit_zentral : Outport  Port=2
  wires:
  Rate Transition21/1 -> Bus Creator1/4  "M_R_ub"
  Rate Transition23/1 -> Bus Creator1/3  "M_R_lb"
  Rate Transition17/1 -> Bus Creator1/2  "M_F_ub"
  Rate Transition19/1 -> Bus Creator1/1  "M_F_lb"
  Bus Creator1/1 -> M_limit_zentral/1
  Gain1/1 -> Rate Transition22/1, Rate Transition20/1
  Add1/1 -> Gain1/1
  Gain/1 -> Rate Transition18/1, Rate Transition16/1
  Add/1 -> Gain/1
  M_Reku5/1 -> Rate Transition23/1
  Rate Transition22/1 -> M_Reku5/1
  M_Antr5/1 -> Rate Transition21/1
  Rate Transition20/1 -> M_Antr5/1
  M_Reku4/1 -> Rate Transition19/1
  Rate Transition18/1 -> M_Reku4/1
  M_Antr4/1 -> Rate Transition17/1
  Rate Transition16/1 -> M_Antr4/1
  Bus Selector/4 -> Rate Transition14/1, Rate Transition12/1, Add1/2  "<omega_RR>"
  Bus Selector/3 -> Rate Transition10/1, Rate Transition8/1, Add1/1  "<omega_LR>"
  M_Reku3/1 -> Rate Transition15/1
  Rate Transition14/1 -> M_Reku3/1
  M_Antr3/1 -> Rate Transition13/1
  Rate Transition12/1 -> M_Antr3/1
  M_Reku2/1 -> Rate Transition9/1
  Rate Transition8/1 -> M_Reku2/1
  M_Antr2/1 -> Rate Transition11/1
  Rate Transition10/1 -> M_Antr2/1
  Bus Selector/2 -> Add/1, Rate Transition4/1, Rate Transition6/1  "<omega_RF>"
  M_Reku1/1 -> Rate Transition5/1
  Rate Transition4/1 -> M_Reku1/1
  M_Antr1/1 -> Rate Transition7/1
  Rate Transition6/1 -> M_Antr1/1
  Bus Selector/1 -> Rate Transition/1, Rate Transition2/1, Add/2  "<omega_LF>"
  Bus Creator/1 -> M_limit/1
  M_Reku/1 -> Rate Transition1/1
  Rate Transition/1 -> M_Reku/1
  M_Antr/1 -> Rate Transition3/1
  Rate Transition2/1 -> M_Antr/1
  Input/1 -> Bus Selector/1
  Rate Transition3/1 -> Bus Creator/2  "M_LF_ub"
  Rate Transition5/1 -> Bus Creator/3  "M_RF_lb"
  Rate Transition7/1 -> Bus Creator/4  "M_RF_ub"
  Rate Transition1/1 -> Bus Creator/1  "M_LF_lb"
  Rate Transition9/1 -> Bus Creator/5  "M_LR_lb"
  Rate Transition11/1 -> Bus Creator/6  "M_LR_ub"
  Rate Transition15/1 -> Bus Creator/7  "M_RR_lb"
  Rate Transition13/1 -> Bus Creator/8  "M_RR_ub"

== system Library_Betriebsstrategie/Momentverteilung_LR2/Radmomentenaufteilung ==
  note: Optimale Distribution Factors
  note: Momentenverteilung
  note: Aufbringen des TV-Moments
  Input : Inport
  M_wheel : Inport  Port=2
  M_z_desired : Inport  Port=3
  Bias : Bias  Bias=-1
  Bias1 : Bias  Bias=-1
  Divide : Product  Inputs=*/
  Divide1 : Product  Inputs=*/
  Gain : Gain  Gain=0.5
  Optimierung links : Subsystem
  Optimierung rechts : Subsystem
  Product{,1..5} (6 alike) : Product
  Scope2 : Scope  NumInputPorts=4
  Sum : Sum  Inputs=|++
  Sum1 : Sum  Inputs=|+-
  To Workspace1 : ToWorkspace  VariableName=sv_M_right  SampleTime=-1
      settings: Decimation=savedec  Save2DSignal=2-D array (concatenate along first dimension)
  To Workspace2 : ToWorkspace  VariableName=sv_M_left  SampleTime=-1
      settings: Decimation=savedec  Save2DSignal=2-D array (concatenate along first dimension)
  To Workspace3 : ToWorkspace  VariableName=sv_gammaL  SampleTime=-1
      settings: Decimation=savedec  Save2DSignal=2-D array (concatenate along first dimension)
  To Workspace4 : ToWorkspace  VariableName=sv_gammaR  SampleTime=-1
      settings: Decimation=savedec  Save2DSignal=2-D array (concatenate along first dimension)
  Unary Minus : UnaryMinus
  Unary Minus1 : UnaryMinus
  r_stat0 : Constant  Value=par_VEH.r_stat0
  sF05 : Constant  Value=par_VEH.sF05
  M_antr_LF : Outport
  M_antr_LR : Outport  Port=2
  M_antr_RF : Outport  Port=3
  M_antr_RR : Outport  Port=4
  wires:
  M_wheel/1 -> Divide/1
  M_z_desired/1 -> Divide1/1
  Divide/1 -> Sum1/1, Sum/1  "F_x"
  Divide1/1 -> Sum1/2, Sum/2
  Sum1/1 -> Product/1
  Gain/1 -> Product1/2, Product/2
  Sum/1 -> Product1/1
  Product/1 -> Optimierung links/1(M_wheel_left), To Workspace2/1, Product5/2, Product3/1  "M_wheel_left"
  Product1/1 -> Optimierung rechts/2(M_wheel_right), To Workspace1/1, Product2/1, Product4/2  "M_wheel_right"
  Product3/1 -> Scope2/1, M_antr_LF/1  "M_LF"
  Product4/1 -> M_antr_RR/1, Scope2/4  "M_RR"
  Product5/1 -> Scope2/2, M_antr_LR/1  "M_LR"
  Optimierung rechts/1(gamma_right) -> To Workspace4/1, Bias1/1, Product2/2
  r_stat0/1 -> Divide/2, Gain/1
  sF05/1 -> Divide1/2
  Product2/1 -> Scope2/3, M_antr_RF/1  "M_RF"
  Input/1 -> Optimierung links/2(Input), Optimierung rechts/1(Input)
  Bias/1 -> Unary Minus/1
  Optimierung links/1(gamma_left) -> To Workspace3/1, Bias/1, Product3/2
  Unary Minus/1 -> Product5/1
  Bias1/1 -> Unary Minus1/1
  Unary Minus1/1 -> Product4/1

== system Library_Betriebsstrategie/Momentverteilung_LR2/Reifen Limits ==
  note: Reifen RF
  note: Reifen LF
  note: Reifen RR
  note: Reifen LR
  note: Für numerische Stabilität
  Input : Inport
  Add{,1..3} (4 alike) : Sum  Inputs=-+
  Bus Creator : BusCreator  Inputs=4
  Bus Selector1 : BusSelector  OutputSignals=Fz.Fz_RF,Fs.Fs_RF,Fz.Fz_LF,Fs.Fs_LF,Fz.Fz_RR,Fs.Fs_RR,Fz.Fz_LR,Fs.Fs_LR
  Constant{,1..3} (4 alike) : Constant
  Constant20 : Constant  Value=mu_road
  Divide{,1..3} (4 alike) : Product  Inputs=/*
  Math Function{,1..3} (4 alike) : Math  Operator=magnitude^2  SaturateOnIntegerOverflow=on
  Product{,1..11} (12 alike) : Product
  Sqrt{,1..3} (4 alike) : Sqrt  SaturateOnIntegerOverflow=on
  Sum{1..4} (4 alike) : Sum  Inputs=|++
  epsilon : Constant  Value=0.0015
  Fx_limit : Outport
  wires:
  epsilon/1 -> Sum2/2, Sum4/2, Sum3/2, Sum1/2
  Sum3/1 -> Product11/2, Product10/2
  Bus Selector1/7 -> Sum3/1  "<Fz_LR>"
  Sum4/1 -> Product8/2, Product9/2
  Bus Selector1/5 -> Sum4/1  "<Fz_RR>"
  Sum2/1 -> Product6/2, Product7/2
  Bus Selector1/3 -> Sum2/1  "<Fz_LF>"
  Sum1/1 -> Product5/2, Product4/2
  Bus Selector1/1 -> Sum1/1  "<Fz_RF>"
  Product4/1 -> Product/1
  Product5/1 -> Divide/1
  Math Function/1 -> Add/1
  Constant/1 -> Add/2
  Add/1 -> Sqrt/1
  Sqrt/1 -> Product/2
  Product8/1 -> Product1/1
  Product9/1 -> Divide1/1
  Divide1/1 -> Math Function1/1
  Math Function1/1 -> Add1/1
  Constant1/1 -> Add1/2
  Add1/1 -> Sqrt1/1
  Sqrt1/1 -> Product1/2
  Product6/1 -> Product2/1
  Product7/1 -> Divide2/1
  Divide2/1 -> Math Function2/1
  Math Function2/1 -> Add2/1
  Constant2/1 -> Add2/2
  Add2/1 -> Sqrt2/1
  Sqrt2/1 -> Product2/2
  Product10/1 -> Product3/1
  Product11/1 -> Divide3/1
  Divide3/1 -> Math Function3/1
  Math Function3/1 -> Add3/1
  Constant3/1 -> Add3/2
  Add3/1 -> Sqrt3/1
  Sqrt3/1 -> Product3/2
  Divide/1 -> Math Function/1
  Input/1 -> Bus Selector1/1
  Constant20/1 -> Product8/1, Product9/1, Product11/1, Product10/1, Product7/1, Product6/1, Product4/1, Product5/1  "mu_road"
  Bus Selector1/2 -> Divide/2  "<Fs_RF>"
  Bus Selector1/4 -> Divide2/2  "<Fs_LF>"
  Bus Selector1/6 -> Divide1/2  "<Fs_RR>"
  Bus Selector1/8 -> Divide3/2  "<Fs_LR>"
  Product/1 -> Bus Creator/1  "FxlimRF"
  Product2/1 -> Bus Creator/2  "FxlimLF"
  Product1/1 -> Bus Creator/3  "FxlimRR"
  Product3/1 -> Bus Creator/4  "FxlimLR"
  Bus Creator/1 -> Fx_limit/1

== system Library_Betriebsstrategie/Inverter Power Input einer Achse/Wirkungsgradberechnung/generatorischer WKG1 ==
  Drehzahl : Inport
  Moment : Inport  Port=2
  Enable : EnablePort
  Abs : Abs
  Saturation : Saturate  UpperLimit=1  LowerLimit=0.05
  Saturation2 : Saturate  UpperLimit=1  LowerLimit=0.2
  Switch : Switch  Criteria=u2 > Threshold  Threshold=120
  Wirkungsgradkennfeld nach Pesce Generatorbetrieb : Lookup_n-D  BreakpointsForDimension1=GeneratorEffMap3D_w  BreakpointsForDimension2=GeneratorEffMap3D_M  Table=GeneratorEffMap3D  UseLastTableValue=on  InternalRulePriority=Speed  RndMeth=Simplest  InputSameDT=on
  WKG : Outport
  wires:
  Saturation2/1 -> Switch/3
  Saturation/1 -> Switch/1
  Drehzahl/1 -> Wirkungsgradkennfeld nach Pesce Generatorbetrieb/1, Switch/2
  Switch/1 -> WKG/1
  Moment/1 -> Abs/1
  Wirkungsgradkennfeld nach Pesce Generatorbetrieb/1 -> Saturation/1, Saturation2/1
  Abs/1 -> Wirkungsgradkennfeld nach Pesce Generatorbetrieb/2

== system Library_Betriebsstrategie/Inverter Power Input einer Achse/Wirkungsgradberechnung/motorischer WKG1 ==
  Drehzahl : Inport
  Moment : Inport  Port=2
  Enable : EnablePort
  Saturation : Saturate  UpperLimit=1  LowerLimit=0.05
  Saturation1 : Saturate  UpperLimit=1  LowerLimit=0.2
  Switch : Switch  Criteria=u2 > Threshold  Threshold=120
  Wirkungsgradkennfeld nach Pesce Motorbetrieb : Lookup_n-D  BreakpointsForDimension1=MotorEffMap3D_w  BreakpointsForDimension2=MotorEffMap3D_M  Table=MotorEffMap3D  UseLastTableValue=on  InternalRulePriority=Speed  RndMeth=Simplest  InputSameDT=on
  WKG : Outport
  wires:
  Saturation1/1 -> Switch/3
  Saturation/1 -> Switch/1
  Switch/1 -> WKG/1
  Drehzahl/1 -> Wirkungsgradkennfeld nach Pesce Motorbetrieb/1, Switch/2
  Moment/1 -> Wirkungsgradkennfeld nach Pesce Motorbetrieb/2
  Wirkungsgradkennfeld nach Pesce Motorbetrieb/1 -> Saturation/1, Saturation1/1

== system Library_Betriebsstrategie/Inverter Power Input einer Achse ALT/Leistungselektronik/Leistungselektronik ==
  Strom : Inport
  Spannung : Inport  Port=2
  Powerfactor : Inport  Port=3
  Add : Sum  Inputs=+-
  Constant : Constant
  Saturation : Saturate  UpperLimit=1  LowerLimit=0.05
  n-D Lookup Table : Lookup_n-D  NumberOfTableDimensions=3  BreakpointsForDimension1=current  BreakpointsForDimension2=voltage  BreakpointsForDimension3=powerfactor  Table=efficiency_map_LE  ExtrapMethod=Clip  UseLastTableValue=on  InternalRulePriority=Speed  RndMeth=Simplest  InputSameDT=on
  "Verlustgrad " : Outport
  wires:
  Saturation/1 -> Add/2
  Constant/1 -> Add/1
  Strom/1 -> n-D Lookup Table/1
  Spannung/1 -> n-D Lookup Table/2
  Powerfactor/1 -> n-D Lookup Table/3
  n-D Lookup Table/1 -> Saturation/1
  Add/1 -> "Verlustgrad "/1

== system Library_Betriebsstrategie/Inverter Power Input einer Achse ALT/Leistungselektronik/Powerfactor ==
  Drehmoment : Inport
  Drehzahl : Inport  Port=2
  2-D Lookup Table : Lookup_n-D  BreakpointsForDimension1=torque  BreakpointsForDimension2=speed  Table=Powerfactor_map  ExtrapMethod=Clip  InternalRulePriority=Speed  RndMeth=Simplest  InputSameDT=on
  Powerfactor : Outport
  wires:
  2-D Lookup Table/1 -> Powerfactor/1
  Drehzahl/1 -> 2-D Lookup Table/2
  Drehmoment/1 -> 2-D Lookup Table/1

== system Library_Betriebsstrategie/Inverter Power Input einer Achse ALT/Leistungselektronik/Strom ==
  Leistung_EM_mech : Inport
  Spannung : Inport  Port=2
  Powerfactor : Inport  Port=3
  Constant : Constant  Value=3
  Divide : Product  Inputs=*///
  Strom : Outport
  wires:
  Divide/1 -> Strom/1
  Leistung_EM_mech/1 -> Divide/1
  Powerfactor/1 -> Divide/4
  Spannung/1 -> Divide/3
  Constant/1 -> Divide/2

== system Library_Betriebsstrategie/Inverter Power Input einer Achse ALT/Wirkungsgradberechnung/generatorischer WKG ==
  Drehzahl : Inport
  Moment : Inport  Port=2
  Enable : EnablePort
  Abs : Abs
  Wirkungsgradkennfeld Generatorbetrieb : Lookup_n-D  BreakpointsForDimension1=GeneratorEffMap3D_w  BreakpointsForDimension2=GeneratorEffMap3D_M  Table=GeneratorEffMap3D  UseLastTableValue=on  InternalRulePriority=Speed  RndMeth=Simplest  InputSameDT=on
  WKG : Outport
  wires:
  Wirkungsgradkennfeld Generatorbetrieb/1 -> WKG/1
  Abs/1 -> Wirkungsgradkennfeld Generatorbetrieb/2
  Moment/1 -> Abs/1
  Drehzahl/1 -> Wirkungsgradkennfeld Generatorbetrieb/1

== system Library_Betriebsstrategie/Inverter Power Input einer Achse ALT/Wirkungsgradberechnung/motorischer WKG ==
  Drehzahl : Inport
  Moment : Inport  Port=2
  Enable : EnablePort
  Wirkungsgradkennfeld Motorbetrieb : Lookup_n-D  BreakpointsForDimension1=MotorEffMap3D_w  BreakpointsForDimension2=MotorEffMap3D_M  Table=MotorEffMap3D  UseLastTableValue=on  InternalRulePriority=Speed  RndMeth=Simplest  InputSameDT=on
  WKG : Outport
  wires:
  Drehzahl/1 -> Wirkungsgradkennfeld Motorbetrieb/1
  Moment/1 -> Wirkungsgradkennfeld Motorbetrieb/2
  Wirkungsgradkennfeld Motorbetrieb/1 -> WKG/1

== system Library_Betriebsstrategie/Momentenverteilung_Diskret/Feedback Controller/Zero Crossing ==
  de0 : Inport
  de1 : Inport  Port=2
  e0 : Inport  Port=3
  e1 : Inport  Port=4
  Product : Product
  Switch : Switch  Criteria=u2 > Threshold
  error(Tc) : Outport
  wires:
  de0/1 -> Product/1
  de1/1 -> Product/2
  Product/1 -> Switch/2
  Switch/1 -> error(Tc)/1
  e1/1 -> Switch/1
  e0/1 -> Switch/3

== system Library_Betriebsstrategie/Momentenverteilung_Fmincon/Feedback Controller/Zero Crossing ==
  de0 : Inport
  de1 : Inport  Port=2
  e0 : Inport  Port=3
  e1 : Inport  Port=4
  Product : Product
  Switch : Switch  Criteria=u2 > Threshold
  error(Tc) : Outport
  wires:
  de0/1 -> Product/1
  de1/1 -> Product/2
  Product/1 -> Switch/2
  Switch/1 -> error(Tc)/1
  e1/1 -> Switch/1
  e0/1 -> Switch/3

== system Library_Betriebsstrategie/Momentenverteilung_Lagrange/Feedback Controller/Zero Crossing ==
  de0 : Inport
  de1 : Inport  Port=2
  e0 : Inport  Port=3
  e1 : Inport  Port=4
  Product : Product
  Switch : Switch  Criteria=u2 > Threshold
  error(Tc) : Outport
  wires:
  de0/1 -> Product/1
  de1/1 -> Product/2
  Product/1 -> Switch/2
  Switch/1 -> error(Tc)/1
  e1/1 -> Switch/1
  e0/1 -> Switch/3

== system Library_Betriebsstrategie/Momentenverteilung_Lagrange1/Feedback Controller/Zero Crossing ==
  de0 : Inport
  de1 : Inport  Port=2
  e0 : Inport  Port=3
  e1 : Inport  Port=4
  Product : Product
  Switch : Switch  Criteria=u2 > Threshold
  error(Tc) : Outport
  wires:
  e0/1 -> Switch/3
  e1/1 -> Switch/1
  Switch/1 -> error(Tc)/1
  Product/1 -> Switch/2
  de1/1 -> Product/2
  de0/1 -> Product/1

== system Library_Betriebsstrategie/Momentenverteilung_Lagrange1/Limitierungen gesamt (mit MVS Limits)/Aktuatoren und Delta TV ==
  Aktuator : Constant  Value=akt_OD_VA
  Aktuator1 : Constant  Value=akt_LSD_VA
  Aktuator2 : Constant  Value=akt_mUELG_VA
  Aktuator3 : Constant  Value=akt_eUELG_VA
  Aktuator4 : Constant  Value=akt_keinMVS_VA
  Aktuator5 : Constant  Value=akt_OD_HA
  Aktuator6 : Constant  Value=akt_LSD_HA
  Aktuator7 : Constant  Value=akt_mUELG_HA
  Aktuator8 : Constant  Value=akt_eUELG_HA
  Aktuator9 : Constant  Value=akt_keinMVS_HA
  Limit elektrisches Überlagerungsgetriebe : Constant  Value=595
  Limit mechanisches Überlagerungsgetriebe1 : Constant  Value=595
  Limit mechanisches Überlagerungsgetriebe2 : Constant  Value=595
  Limit mechanisches Überlagerungsgetriebe3 : Constant  Value=595
  TV Moment pro Achse : MATLAB Function  TreatAsAtomicUnit=on
  Zuweisung Aktuatoren : MATLAB Function  TreatAsAtomicUnit=on
  Delta_T_f : Outport
  Delta_T_r : Outport  Port=2
  A_f : Outport  Port=3
  A_r : Outport  Port=4
  wires:
  Zuweisung Aktuatoren/1(a_f) -> A_f/1, TV Moment pro Achse/6(a_f)
  Aktuator9/1 -> Zuweisung Aktuatoren/10(A10)
  Aktuator8/1 -> Zuweisung Aktuatoren/9(A9)
  Aktuator7/1 -> Zuweisung Aktuatoren/8(A8)
  Aktuator6/1 -> Zuweisung Aktuatoren/7(A7)
  Aktuator5/1 -> Zuweisung Aktuatoren/6(A6)
  Aktuator4/1 -> Zuweisung Aktuatoren/5(A5)
  Aktuator3/1 -> Zuweisung Aktuatoren/4(A4)
  Aktuator2/1 -> Zuweisung Aktuatoren/3(A3)
  Aktuator1/1 -> Zuweisung Aktuatoren/2(A2)
  Aktuator/1 -> Zuweisung Aktuatoren/1(A1)
  Zuweisung Aktuatoren/2(a_r) -> A_r/1, TV Moment pro Achse/7(a_r)
  TV Moment pro Achse/1(Delta_T_f) -> Delta_T_f/1
  TV Moment pro Achse/2(Delta_T_r) -> Delta_T_r/1
  Limit elektrisches Überlagerungsgetriebe/1 -> TV Moment pro Achse/1(L1)
  Limit mechanisches Überlagerungsgetriebe1/1 -> TV Moment pro Achse/2(L2)
  Limit mechanisches Überlagerungsgetriebe2/1 -> TV Moment pro Achse/3(L3)
  Limit mechanisches Überlagerungsgetriebe3/1 -> TV Moment pro Achse/4(L4)

== system Library_Betriebsstrategie/Momentenverteilung_Lagrange2/Feedback Controller/Zero Crossing ==
  de0 : Inport
  de1 : Inport  Port=2
  e0 : Inport  Port=3
  e1 : Inport  Port=4
  Product : Product
  Switch : Switch  Criteria=u2 > Threshold
  error(Tc) : Outport
  wires:
  de0/1 -> Product/1
  de1/1 -> Product/2
  Product/1 -> Switch/2
  Switch/1 -> error(Tc)/1
  e1/1 -> Switch/1
  e0/1 -> Switch/3
